simulink model "LMPC_ay_r_step_sinus"  (R2019a)
settings: Solver=FixedStepAuto  StartTime=0.0  StopTime=10.0  RelTol=1e-3
undefined symbols (not defined in the file): Cf, Cr, Iz, lf, lr, m
libraries: mpclib x2
settings Model: Creator=Johan PC  LastModifiedBy=Johan PC
settings DataIOCC: ReturnWorkspaceOutputs=off
settings OptimizationCC: DefaultParameterBehavior=Inlined  EnhancedBackFolding=on  PassReuseOutputArgsAs=Individual arguments  OptimizeBlockOrder=speed  DifferentSizesBufferReuse=on
settings DebuggingCC: ParameterTunabilityLossMsg=error  ArithmeticOperatorsInVariantConditions=warning
settings SFSimCC: MATLABDynamicMemAlloc=off
settings RTWCC: SystemTargetFile=ert.tlc  TemplateMakefile=ert_default_tmf  GenerateReport=on  IncludeHyperlinkInReport=on  LaunchReport=on  GenerateTraceInfo=on  GenerateTraceReport=on  GenerateTraceReportSl=on  GenerateTraceReportSf=on  GenerateTraceReportEml=on
settings CodeAppCC: ForceParamTrailComments=on  IgnoreCustomStorageClasses=off  OperatorAnnotations=on  SimulinkDataObjDesc=on  SFDataObjDesc=on  InsertBlockDesc=on
settings ERTTargetCC: TargetLangStandard=C99 (ISO)  GenerateSampleERTMain=on  InlinedParameterPlacement=NonHierarchical  RTWCAPISignals=on  ERTCustomFileTemplate=example_file_process.tlc

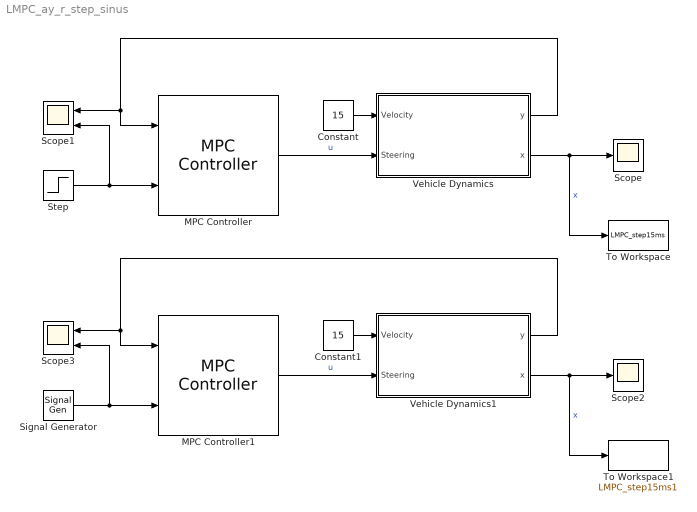
== system LMPC_ay_r_step_sinus ==
  Constant : Constant  Value=15
  Constant1 : Constant  Value=15
  MPC Controller : mpclib/MPC Controller  SCDEnableBlockLinearizationSpecification=on  mpcobj=mpc1  is_multiple=0  enable_value=0  return_u0=off  updateMPCinCallerWorkspace=on  md_inport=off  mv_inport=off  uref_inport=off  return_cost=off  return_mvseq=off  return_qpstatus=off  return_xseq=off  return_state=off  return_ovseq=off  state_inport=off  umin_inport=off  umax_inport=off  ymin_inport=off  ymax_inport=off  cc_inport=off  ywt_inport=off  uwt_inport=off  duwt_inport=off  rhoeps_inport=off  pm_inport=off  MaximumP=10  HorizonChoice=FixedHorizon  n_ts=0.001  n_p=10  n_mv=1  n_md=0  n_ud=0  n_mo=2  n_uo=0  BlockDataType=double  SampleTimeInherited=off  switch_inport=off
  MPC Controller1 : mpclib/MPC Controller  SCDEnableBlockLinearizationSpecification=on  mpcobj=mpc1  is_multiple=0  enable_value=0  return_u0=off  updateMPCinCallerWorkspace=on  md_inport=off  mv_inport=off  uref_inport=off  return_cost=off  return_mvseq=off  return_qpstatus=off  return_xseq=off  return_state=off  return_ovseq=off  state_inport=off  umin_inport=off  umax_inport=off  ymin_inport=off  ymax_inport=off  cc_inport=off  ywt_inport=off  uwt_inport=off  duwt_inport=off  rhoeps_inport=off  pm_inport=off  MaximumP=10  HorizonChoice=FixedHorizon  n_ts=0.001  n_p=10  n_mv=1  n_md=0  n_ud=0  n_mo=2  n_uo=0  BlockDataType=double  SampleTimeInherited=off  switch_inport=off
  Scope : Scope
  Scope1 : Scope  NumInputPorts=2
  Scope2 : Scope
  Scope3 : Scope  NumInputPorts=2
  Signal Generator : SignalGenerator  Frequency=2  Units=rad/sec
  Step : Step  Time=0.5  SampleTime=0
  To Workspace : ToWorkspace  VariableName=LMPC_step15ms  SaveFormat=Timeseries  SampleTime=0.01
  To Workspace1 : ToWorkspace  VariableName=LMPC_step15ms1  SaveFormat=Timeseries  SampleTime=0.01
  Vehicle Dynamics : Subsystem
  Vehicle Dynamics1 : Subsystem
  wires:
  MPC Controller/1 -> Vehicle Dynamics/2(Steering)  "u"
  Step/1 -> MPC Controller/2, Scope1/2
  Constant/1 -> Vehicle Dynamics/1(Velocity)
  Vehicle Dynamics/2(x) -> To Workspace/1, Scope/1  "x"
  Vehicle Dynamics/1("y ") -> Scope1/1, MPC Controller/1
  Vehicle Dynamics1/1("y ") -> MPC Controller1/1, Scope3/1
  Vehicle Dynamics1/2(x) -> Scope2/1, To Workspace1/1  "x"
  Constant1/1 -> Vehicle Dynamics1/1(Velocity)
  Signal Generator/1 -> Scope3/2, MPC Controller1/2
  MPC Controller1/1 -> Vehicle Dynamics1/2(Steering)  "u"

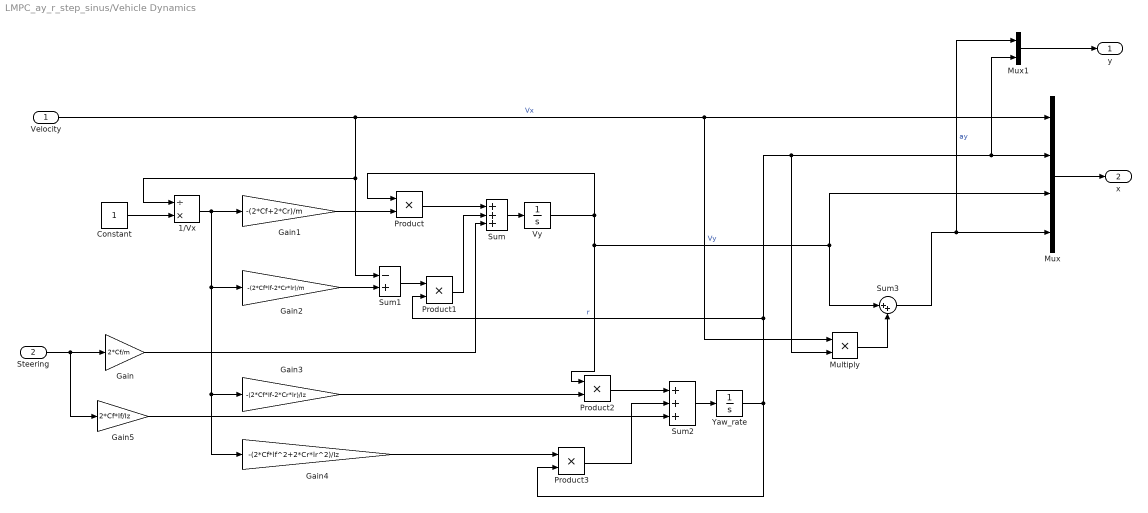
== system LMPC_ay_r_step_sinus/Vehicle Dynamics ==
  Velocity : Inport
  Steering : Inport  Port=2
  1/Vx : Product  Inputs=/*
  Constant : Constant
  Gain : Gain  Gain=2*Cf/m
  Gain1 : Gain  Gain=-(2*Cf+2*Cr)/m
  Gain2 : Gain  Gain=-(2*Cf*lf-2*Cr*lr)/m
  Gain3 : Gain  Gain=-(2*Cf*lf-2*Cr*lr)/Iz
  Gain4 : Gain  Gain=-(2*Cf*lf^2+2*Cr*lr^2)/Iz
  Gain5 : Gain  Gain=2*Cf*lf/Iz
  Multiply : Product
  Mux : Mux
  Mux1 : Mux  Inputs=2
  Product{,1..3} (4 alike) : Product
  Sum : Sum  Inputs=+++
  Sum1 : Sum  Inputs=-+
  Sum2 : Sum  Inputs=+++
  Sum3 : Sum  Inputs=|++
  Vy : Integrator
  "Yaw_rate " : Integrator
  "y " : Outport
  x : Outport  Port=2
  wires:
  Sum2/1 -> "Yaw_rate "/1
  Gain2/1 -> Sum1/2
  Gain4/1 -> Product3/1
  Constant/1 -> 1/Vx/2
  Gain3/1 -> Product2/2
  1/Vx/1 -> Gain4/1, Gain3/1, Gain2/1, Gain1/1
  Product2/1 -> Sum2/1
  Product3/1 -> Sum2/2
  Gain5/1 -> Sum2/3
  Sum1/1 -> Product1/1
  "Yaw_rate "/1 -> Multiply/2, Mux1/2, Mux/2, Product1/2, Product3/2  "r"
  Gain/1 -> Sum/3
  Steering/1 -> Gain/1, Gain5/1
  Gain1/1 -> Product/2
  Product/1 -> Sum/1
  Vy/1 -> Product2/1, Mux/3, Sum3/1, Product/1  "Vy"
  Sum/1 -> Vy/1
  Velocity/1 -> Mux/1, Multiply/1, 1/Vx/1, Sum1/1  "Vx"
  Product1/1 -> Sum/2
  Multiply/1 -> Sum3/2
  Sum3/1 -> Mux1/1, Mux/4  "ay"
  Mux/1 -> x/1
  Mux1/1 -> "y "/1

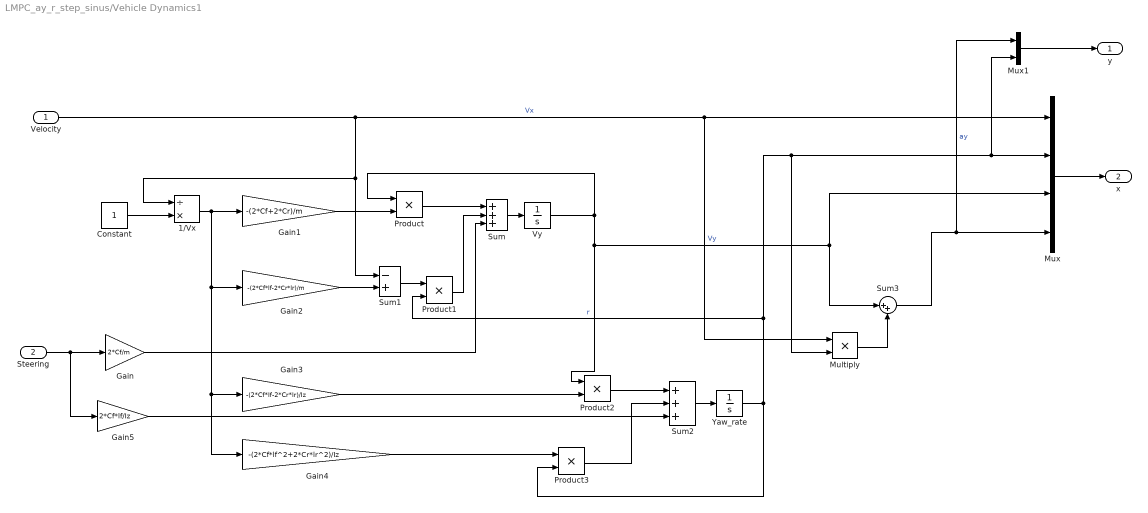
== system LMPC_ay_r_step_sinus/Vehicle Dynamics1 ==
  Velocity : Inport
  Steering : Inport  Port=2
  1/Vx : Product  Inputs=/*
  Constant : Constant
  Gain : Gain  Gain=2*Cf/m
  Gain1 : Gain  Gain=-(2*Cf+2*Cr)/m
  Gain2 : Gain  Gain=-(2*Cf*lf-2*Cr*lr)/m
  Gain3 : Gain  Gain=-(2*Cf*lf-2*Cr*lr)/Iz
  Gain4 : Gain  Gain=-(2*Cf*lf^2+2*Cr*lr^2)/Iz
  Gain5 : Gain  Gain=2*Cf*lf/Iz
  Multiply : Product
  Mux : Mux
  Mux1 : Mux  Inputs=2
  Product{,1..3} (4 alike) : Product
  Sum : Sum  Inputs=+++
  Sum1 : Sum  Inputs=-+
  Sum2 : Sum  Inputs=+++
  Sum3 : Sum  Inputs=|++
  Vy : Integrator
  "Yaw_rate " : Integrator
  "y " : Outport
  x : Outport  Port=2
  wires:
  Mux1/1 -> "y "/1
  Mux/1 -> x/1
  Sum3/1 -> Mux/4, Mux1/1  "ay"
  Multiply/1 -> Sum3/2
  Product1/1 -> Sum/2
  Velocity/1 -> Sum1/1, 1/Vx/1, Multiply/1, Mux/1  "Vx"
  Sum/1 -> Vy/1
  Vy/1 -> Product/1, Sum3/1, Mux/3, Product2/1  "Vy"
  Product/1 -> Sum/1
  Gain1/1 -> Product/2
  Steering/1 -> Gain5/1, Gain/1
  Gain/1 -> Sum/3
  "Yaw_rate "/1 -> Product3/2, Product1/2, Mux/2, Mux1/2, Multiply/2  "r"
  Sum1/1 -> Product1/1
  Gain5/1 -> Sum2/3
  Product3/1 -> Sum2/2
  Product2/1 -> Sum2/1
  1/Vx/1 -> Gain1/1, Gain2/1, Gain3/1, Gain4/1
  Gain3/1 -> Product2/2
  Constant/1 -> 1/Vx/2
  Gain4/1 -> Product3/1
  Gain2/1 -> Sum1/2
  Sum2/1 -> "Yaw_rate "/1
